simulink model "DiscreteTransferFcn_2_orig_vs_preprocessed"  (R2017b)
settings: Solver=FixedStepAuto  StartTime=0.0  StopTime=10.0  FixedStep=0.100000  RelTol=1e-3  EnableMultiTasking=on
model workspace (MAT data in the model file):
  already_pp = 0
  input_struct.time = [0; 0.2; 0.4; 0.6; 0.8; 1; 1.2; 1.4; 1.6; 1.8; 2; 2.2; 2.4; 2.6; 2.8; 3; 3.2; 3.4; 3.6; 3.8; 4; 4.2; 4.4; 4.6; 4.8; 5; 5.2; 5.4; 5.6; 5.8; 6; 6.2; 6.4; 6.6; 6.8; 7; 7.2; 7.4; 7.6; 7.8; 8; 8.2; 8.4; 8.6; 8.8; 9; 9.2; 9.4; 9.6; 9.8; 10; 10.2; 10.4; 10.6; 10.8; 11; 11.2; 11.4; 11.6; 11.8; 12; 12.2; 12.4; 12.6; 12.8; 13; 13.2; 13.4; 13.6; 13.8; 14; 14.2; 14.4; 14.6; 14.8; 15; 15.2; 15.4; 15.6; 15.8; 16; 16.2; 16.4; 16.6; 16.8; 17; 17.2; 17.4; 17.6; 17.8; 18; 18.2; 18.4; 18.6; 18.8; 19; 19.2; 19.4; 19.6; 19.8]
  input_struct.signals.name = 'In1'
  input_struct.signals.values = [62.9447372786; 81.1583874151; -74.6026367413; 82.6751712278; 26.4718492451; -80.4919190001; -44.3003562266; 9.376303841; 91.5013670869; 92.9777070399; -68.4773836645; 94.1185563521; 91.4333896486; -2.92487025543; 60.0560937778; -71.6227322746; -15.6477434747; 83.1471050378; 58.4414659119; 91.8984852786; 31.1481398313; -92.8576642852; 69.8258611738; 86.7986495515; 35.7470309716; 51.5480261157; 48.626493625; -21.5545960932; 31.0955780355; -65.7626624377; 41.2092176039; -93.6334307245; -44.6154030078; -90.7657218738; -80.5736437528; 64.6915656655; 38.9657245952; -36.5801039878; 90.0444097677; -93.1107838994; -12.2511280687; -23.6883085814; 53.1033576298; 59.0399802274; -62.6254790891; -2.04712084235; -10.8827598578; 29.2626020223; 41.8729661716; 50.9373363965; -44.7949846003; 35.9405353707; 31.0196007948; -67.4776529611; -76.2004636883; -0.327189603571; 91.9487917032; -31.9228546668; 17.053550196; -55.2376121018; 50.2534118611; -48.9809769081; 1.19141033303; 39.8153445313; 78.1806505072; 91.8582850411; 9.44310599276; -72.2751114343; -70.1411988882; -48.4983491753; 68.1434511967; -49.1435642057; 62.8569652138; -51.295006255; 85.8527246374; -30.003246803; -60.6809499138; -49.7832284048; 23.2089352293; -5.34223021945; -29.6680985874; 66.1657255793; 17.0528182305; 9.94472165823; 83.438732766; -42.8321962359; 51.4400458221; 50.7458188557; -23.9108306049; 13.564328145; -84.8291420874; -89.2099762667; 6.15951060179; 55.8334460204; 86.8021368458; -74.0187583053; 13.7647321744; -6.12187178836; -97.6195860998; -32.5754711202]
  input_struct.signals.dimensions = 1
settings Model: Creator=arnaud  LastModifiedBy=hbourbou
settings DataIOCC: LimitDataPoints=on  SaveFormat=Structure  SignalLoggingSaveFormat=ModelDataLogs
settings OptimizationCC: ExpressionDepthLimit=2147483647  LifeSpan=inf
settings DebuggingCC: UnderspecifiedInitializationDetection=Classic  MergeDetectMultiDrivingBlocksExec=none  SolverPrmCheckMsg=warning  FcnCallInpInsideContextMsg=warning  StateNameClashWarn=warning  SFUnexpectedBacktrackingDiag=warning  SFNoUnconditionalDefaultTransitionDiag=warning  SFExecutionAtInitializationDiag=none
settings HardwareCC: ProdBitPerPointer=32  ProdBitPerSizeT=32  ProdBitPerPtrDiffT=32  ProdLargestAtomicFloat=None  ProdIntDivRoundTo=Undefined  ProdEndianess=Unspecified  ProdWordSize=32  ProdHWDeviceType=32-bit Generic
settings ModelReferenceCC: PropagateSignalLabelsOutOfModel=off
settings CodeAppCC: StateflowObjectComments=on
settings GRTTargetCC: TargetLangStandard=C89/C90 (ANSI)  GeneratePreprocessorConditionals=Disable all  CombineOutputUpdateFcns=off  GRTInterface=on
settings ConfigComp: CovMetricSettings=dw  CovHtmlReporting=on  CovSaveCumulativeToWorkspaceVar=on  CovSaveSingleToWorkspaceVar=on  CovExternalEMLEnable=off  CovSFcnEnable=off

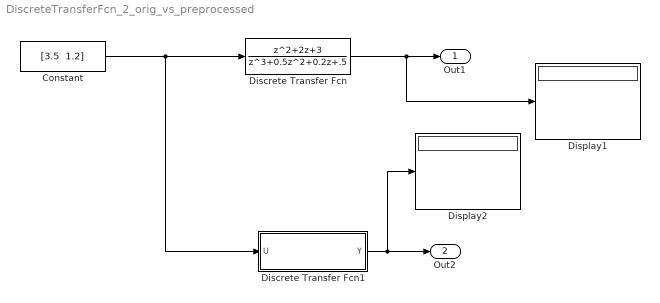
== system DiscreteTransferFcn_2_orig_vs_preprocessed ==
  Constant : Constant  Value="[3.5  1.2]"
  Discrete Transfer Fcn : DiscreteTransferFcn  Numerator=[1 2 3 ]  Denominator=[1 0.5 0.2 .5]  SampleTime=.1
  Discrete Transfer Fcn1 : Subsystem  TreatAsAtomicUnit=on
      settings: MinAlgLoopOccurrences=on
  Display1 : Display
  Display2 : Display
  Out1 : Outport
  Out2 : Outport  Port=2
  wires:
  Discrete Transfer Fcn/1 -> Display1/1, Out1/1
  Constant/1 -> Discrete Transfer Fcn1/1(U), Discrete Transfer Fcn/1
  Discrete Transfer Fcn1/1(Y) -> Display2/1, Out2/1

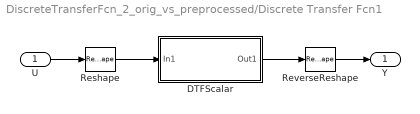
== system DiscreteTransferFcn_2_orig_vs_preprocessed/Discrete Transfer Fcn1 ==
  U : Inport
  DTFScalar : Subsystem  TreatAsAtomicUnit=on
      settings: MinAlgLoopOccurrences=on
  Reshape : Reshape  OutputDimensionality=Column vector (2-D)
  ReverseReshape : Reshape  OutputDimensionality=Customize  OutputDimensions=[2 1]
  Y : Outport
  wires:
  ReverseReshape/1 -> Y/1
  Reshape/1 -> DTFScalar/1(In1)
  DTFScalar/1(Out1) -> ReverseReshape/1
  U/1 -> Reshape/1

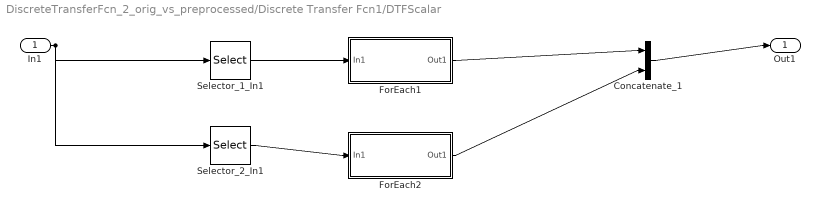
== system DiscreteTransferFcn_2_orig_vs_preprocessed/Discrete Transfer Fcn1/DTFScalar ==
  In1 : Inport
  Concatenate_1 : Concatenate  Mode=Multidimensional array
  ForEach1 : Subsystem  TreatAsAtomicUnit=on
      settings: MinAlgLoopOccurrences=on
  ForEach2 : Subsystem  TreatAsAtomicUnit=on
      settings: MinAlgLoopOccurrences=on
  Selector_1_In1 : Selector  NumberOfDimensions=2  IndexOptions=Index vector (dialog),Select all  Indices=1,  OutputSizes=1
  Selector_2_In1 : Selector  NumberOfDimensions=2  IndexOptions=Index vector (dialog),Select all  Indices=2,  OutputSizes=1
  Out1 : Outport
  wires:
  Concatenate_1/1 -> Out1/1
  ForEach2/1(Out1) -> Concatenate_1/2
  Selector_2_In1/1 -> ForEach2/1(In1)
  ForEach1/1(Out1) -> Concatenate_1/1
  Selector_1_In1/1 -> ForEach1/1(In1)
  In1/1 -> Selector_2_In1/1, Selector_1_In1/1

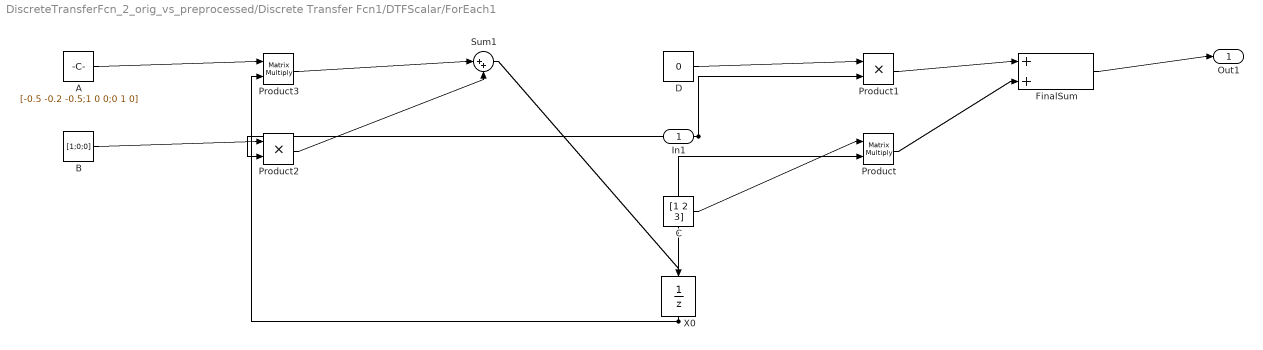
== system DiscreteTransferFcn_2_orig_vs_preprocessed/Discrete Transfer Fcn1/DTFScalar/ForEach1 ==
  In1 : Inport
  A : Constant  Value=[-0.5 -0.2 -0.5;1 0 0;0 1 0]  VectorParams1D=off
  B : Constant  Value=[1;0;0]  VectorParams1D=off
  C : Constant  Value=[1 2 3]  VectorParams1D=off
  D : Constant  Value=0  VectorParams1D=off
  FinalSum : Sum  Inputs=|++
  Product : Product  Multiplication=Matrix(*)
  Product1 : Product
  Product2 : Product
  Product3 : Product  Multiplication=Matrix(*)
  Sum1 : Sum  Inputs=|++
  X0 : UnitDelay  SampleTime=.1
  Out1 : Outport
  wires:
  FinalSum/1 -> Out1/1
  Product/1 -> FinalSum/2
  X0/1 -> Product3/2, Product/2
  Sum1/1 -> X0/1
  Product2/1 -> Sum1/2
  B/1 -> Product2/1
  Product3/1 -> Sum1/1
  A/1 -> Product3/1
  C/1 -> Product/1
  Product1/1 -> FinalSum/1
  In1/1 -> Product2/2, Product1/2
  D/1 -> Product1/1

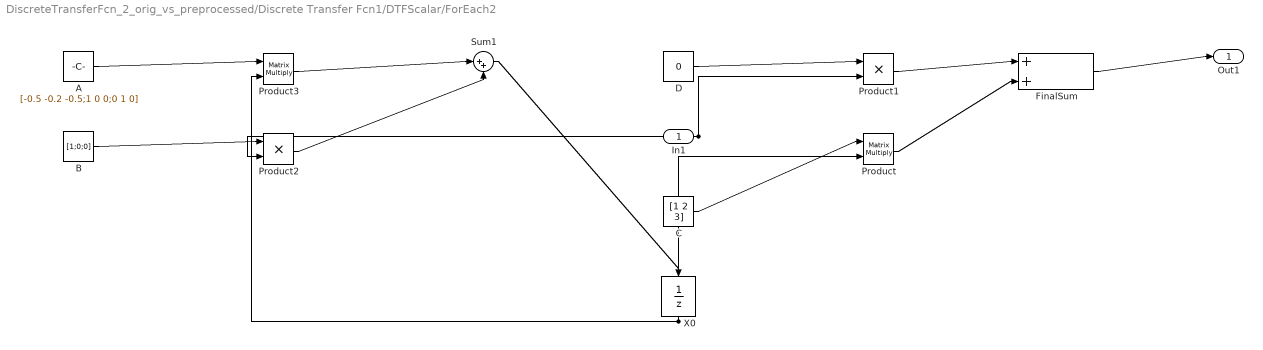
== system DiscreteTransferFcn_2_orig_vs_preprocessed/Discrete Transfer Fcn1/DTFScalar/ForEach2 ==
  In1 : Inport
  A : Constant  Value=[-0.5 -0.2 -0.5;1 0 0;0 1 0]  VectorParams1D=off
  B : Constant  Value=[1;0;0]  VectorParams1D=off
  C : Constant  Value=[1 2 3]  VectorParams1D=off
  D : Constant  Value=0  VectorParams1D=off
  FinalSum : Sum  Inputs=|++
  Product : Product  Multiplication=Matrix(*)
  Product1 : Product
  Product2 : Product
  Product3 : Product  Multiplication=Matrix(*)
  Sum1 : Sum  Inputs=|++
  X0 : UnitDelay  SampleTime=.1
  Out1 : Outport
  wires:
  FinalSum/1 -> Out1/1
  Product/1 -> FinalSum/2
  X0/1 -> Product3/2, Product/2
  Sum1/1 -> X0/1
  Product2/1 -> Sum1/2
  B/1 -> Product2/1
  Product3/1 -> Sum1/1
  A/1 -> Product3/1
  C/1 -> Product/1
  Product1/1 -> FinalSum/1
  In1/1 -> Product2/2, Product1/2
  D/1 -> Product1/1
